simulink model "SlipEstimation"  (R2020b)
settings: Solver=VariableStepAuto  StartTime=0.0  StopTime=10.0  RelTol=1e-3
settings Model: Creator=Authorized User  LastModifiedBy=Authorized User

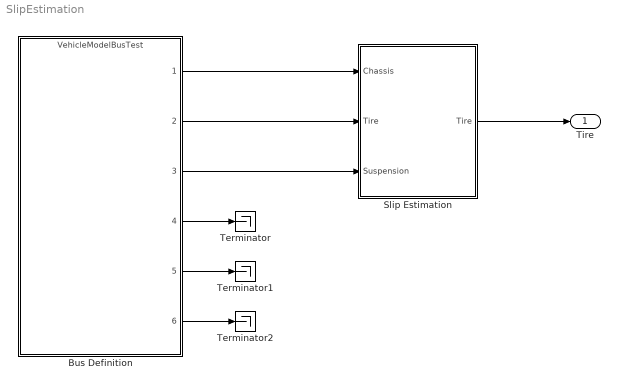
== system SlipEstimation ==
  Bus Definition : ModelReference  ModelNameDialog=VehicleModelBusTest.slx  SimulationMode=Normal  ModelReferenceVersion=1.30
  Slip Estimation : MATLAB Function  TreatAsAtomicUnit=on
  Terminator : Terminator
  Terminator1 : Terminator
  Terminator2 : Terminator
  Tire : Outport
  wires:
  Bus Definition/4 -> Terminator/1
  Bus Definition/5 -> Terminator1/1
  Bus Definition/6 -> Terminator2/1
  Bus Definition/1 -> Slip Estimation/1(Chassis)
  Bus Definition/3 -> Slip Estimation/3(Suspension)
  Bus Definition/2 -> Slip Estimation/2("Tire ")
  Slip Estimation/1(Tire) -> Tire/1

== matlab function SlipEstimation/Slip Estimation ==
  data: Chassis input Bus: Chassis; Tire input Bus: Tire; Suspension input Bus: Suspension; Tire output; Vehicle parameter
function Tire = SlipEstimation(Chassis, Tire, Suspension, Vehicle)
%% Calculate Slip Angle
Tire.Slip_Angle(1) = Suspension.Steer(1) - atan2d( ...
    Chassis.Lateral(2) + Vehicle.Suspension.a*Chassis.Yaw(2), ...
    Chassis.Longitudinal(2) - Suspension.Track(1)*Chassis.Yaw(2) );

Tire.Slip_Angle(2) = Suspension.Steer(2) - atan2d( ...
    Chassis.Lateral(2) + Vehicle.Suspension.a*Chassis.Yaw(2), ...
    Chassis.Longitudinal(2) + Suspension.Track(1)*Chassis.Yaw(2) );

Tire.Slip_Angle(3) = Suspension.Steer(3) - atan2d( ...
    Chassis.Lateral(2) - Vehicle.Suspension.b*Chassis.Yaw(2), ...
    Chassis.Longitudinal(2) - Suspension.Track(3)*Chassis.Yaw(2) );

Tire.Slip_Angle(4) = Suspension.Steer(4) - atan2d( ...
    Chassis.Lateral(2) - Vehicle.Suspension.b*Chassis.Yaw(2), ...
    Chassis.Longitudinal(2) + Suspension.Track(4)*Chassis.Yaw(2) );

%% Tire Center Velocity
vt = zeros(4,1);
vt(1) = sqrt( ( Chassis.Longitudinal(2) - (Suspension.Track(1))*Chassis.Yaw(2) )^2 + ...
    ( Chassis.Lateral(2) + Vehicle.Suspension.a*Chassis.Yaw(2) )^2 );
vt(2) = sqrt( ( Chassis.Longitudinal(2) + (Suspension.Track(1))*Chassis.Yaw(2) )^2 + ...
    ( Chassis.Lateral(2) + Vehicle.Suspension.a*Chassis.Yaw(2) )^2 );
vt(3) = sqrt( ( Chassis.Longitudinal(2) - (Suspension.Track(1))*Chassis.Yaw(2) )^2 + ...
    ( Chassis.Lateral(2) - Vehicle.Suspension.b*Chassis.Yaw(2) )^2 );
vt(4) = sqrt( ( Chassis.Longitudinal(2) + (Suspension.Track(1))*Chassis.Yaw(2) )^2 + ...
    ( Chassis.Lateral(2) - Vehicle.Suspension.b*Chassis.Yaw(2) )^2 );

%% Calculate Slip Ratio
for i = 1:4
    if vt(i) == 0
        Tire.Slip_Ratio(i) = 0;
    else
        Tire.Slip_Ratio(i) = ( Tire.Spin_Rate(i) .* Tire.Effective_Radius(i) ) ./ ...
            ( vt(i) .* cosd(Tire.Slip_Angle(i)) ) - 1;
    end
end
